simulink model "lqi16_discreto"  (R2025b)
settings: Solver=VariableStepAuto  StartTime=0.0  StopTime=10  RelTol=1e-3
values from neighbouring files (symbols this model uses):
  Cm = [1 0 0 0 0 0 0 0 0 0 1 0 ... (108 elements, 9x12)]    [parametros_LQI.mat]
  K = [8.61388977208e-09 -3.23938755891e-11 27.1624608635 1.22408347835e-11 5.15548702544e-09 -26.9052309444 4.91703547324e-11 2.27757364143e-13 56.1282376315 -9.6103215742e-14 8.73666069887e-14 -5.56559839576e-15 ... (64 elements, 4x16)]    [parametros_LQI.mat]
undefined symbols (not defined in the file or in its folder): C, L, sys
settings Model: Creator=rel  LastModifiedBy=rel

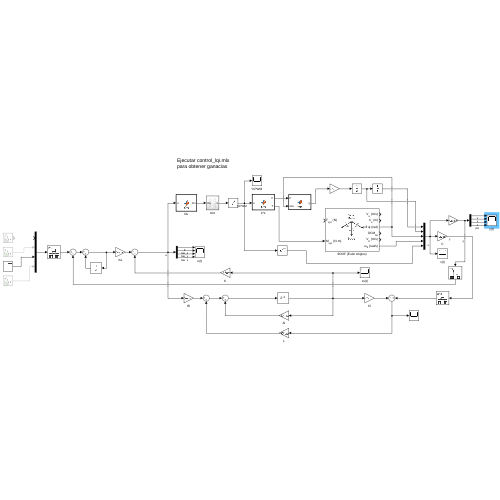
[thumbnail: Simulink's stored preview of the top-level diagram]
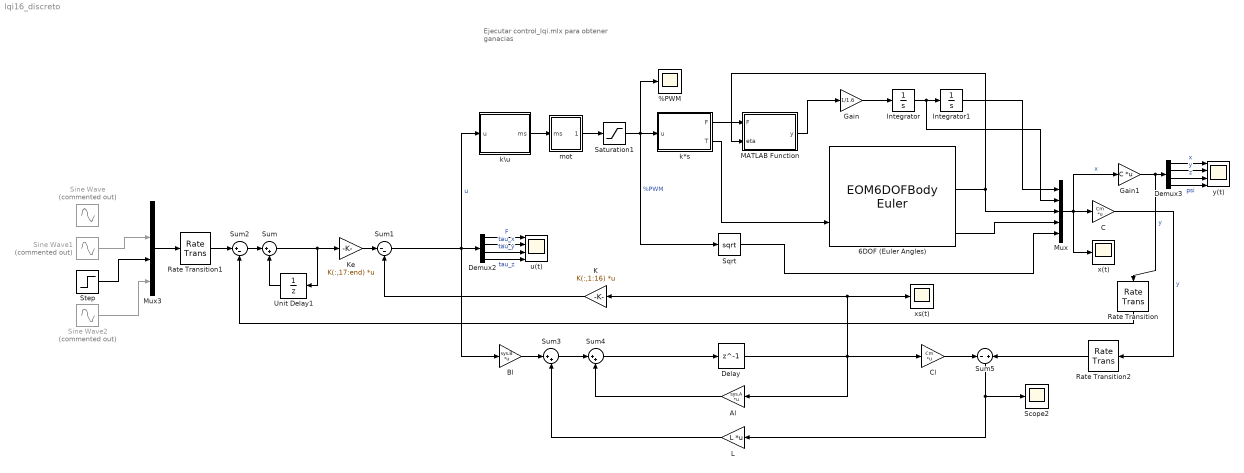
== system lqi16_discreto ==
  note: Ejecutar control_lqi.mlx
      | para obtener ganacias
  %PWM : Scope
      settings: ActiveDisplayYMinimum=-1  ActiveDisplayYMaximum=1  DataLoggingVariableName=ScopeData4
  6DOF (Euler Angles) : EOM6DOFBodyEuler  mass_0=1.6  inertia=diag([0.021915027 0.022124548 0.042349865])
  Al : Gain  Gain=sys.A  Multiplication=Matrix(K*u) (u vector)
  Bl : Gain  Gain=sys.B  Multiplication=Matrix(K*u) (u vector)
  C : Gain  Gain=Cm  Multiplication=Matrix(K*u) (u vector)
  Cl : Gain  Gain=Cm  Multiplication=Matrix(K*u)
  Delay : Delay  DelayLength=1
  Demux2 : Demux
  Demux3 : Demux
  Gain : Gain  Gain=1/1.6
  Gain1 : Gain  Gain=C  Multiplication=Matrix(K*u) (u vector)
  Integrator : Integrator
  Integrator1 : Integrator
  K : Gain  Gain=K(:,1:16)  Multiplication=Matrix(K*u) (u vector)
  Ke : Gain  Gain=K(:,17:end)  Multiplication=Matrix(K*u) (u vector)
  L : Gain  Gain=L  Multiplication=Matrix(K*u) (u vector)
  MATLAB Function : MATLAB Function  TreatAsAtomicUnit=on
  Mux : Mux  Inputs=5
  Mux3 : Mux
  Rate Transition : RateTransition  OutPortSampleTime=1/100
  Rate Transition1 : RateTransition  OutPortSampleTime=1/100
  Rate Transition2 : RateTransition  OutPortSampleTime=1/100
  Saturation1 : Saturate  UpperLimit=1  LowerLimit=0
  Scope2 : Scope
      settings: ActiveDisplayYMinimum=-1  ActiveDisplayYMaximum=1  DataLoggingVariableName=ScopeData6
  Sine Wave : Sin  Commented=on  Amplitude=0.5  Bias=1  Frequency=2  SampleTime=0
  Sine Wave1 : Sin  Commented=on  Amplitude=0.3  Frequency=3  SampleTime=0
  Sine Wave2 : Sin  Commented=on  SampleTime=0
  Sqrt : Sqrt
  Step : Step  SampleTime=0
  Sum : Sum  Inputs=|++
  Sum1 : Sum  Inputs=|--
  Sum2 : Sum  Inputs=|+-
  Sum3 : Sum  Inputs=|++
  Sum4 : Sum  Inputs=|++
  Sum5 : Sum  Inputs=-|+
  Unit Delay1 : UnitDelay  SampleTime=1/100  HasFrameUpgradeWarning=on
  k*s : MATLAB Function  TreatAsAtomicUnit=on
  k\u : MATLAB Function  TreatAsAtomicUnit=on
  mot : Subsystem
  u(t) : Scope  NumInputPorts=4
      settings: ActiveDisplayYMinimum=-47.245581502984457  ActiveDisplayYMaximum=52.593265856388996
  x(t) : Scope
      settings: ActiveDisplayYMinimum=-6.1052768376848006  ActiveDisplayYMaximum=6.0749182298943305  DataLoggingVariableName=ScopeData3
  xs(t) : Scope
      settings: ActiveDisplayYMinimum=-1  ActiveDisplayYMaximum=1  DataLoggingVariableName=ScopeData7
  y(t) : Scope  NumInputPorts=4
      settings: ActiveDisplayYMinimum=-326.12791447062108  ActiveDisplayYMaximum=63.895398333453315
  wires:
  Gain1/1 -> Rate Transition/1, Demux3/1  "y"
  K/1 -> Sum1/2
  Sum/1 -> Ke/1, Unit Delay1/1
  6DOF (Euler Angles)/3 -> MATLAB Function/2(eta), Mux/3
  mot/1(Out1) -> Saturation1/1
  k\u/1(ms) -> mot/1(ms)
  Saturation1/1 -> Sqrt/1, %PWM/1, k*s/1(u)  "%PWM"
  k*s/2(T) -> 6DOF (Euler Angles)/2
  k*s/1(F) -> MATLAB Function/1(F)
  Bl/1 -> Sum3/1
  Sum3/1 -> Sum4/1
  Cl/1 -> Sum5/1
  Al/1 -> Sum4/2
  L/1 -> Sum3/2
  Sum5/1 -> L/1, Scope2/1
  Integrator/1 -> Mux/2, Integrator1/1
  6DOF (Euler Angles)/6 -> Mux/4
  Mux/1 -> Gain1/1, x(t)/1, C/1  "x"
  Unit Delay1/1 -> Sum/2
  Sum2/1 -> Sum/1
  Ke/1 -> Sum1/1
  Mux3/1 -> Rate Transition1/1
  Sum1/1 -> Bl/1, Demux2/1, k\u/1(u)  "u"
  Sine Wave1/1 -> Mux3/2
  Sine Wave2/1 -> Mux3/4
  Demux2/1 -> u(t)/1  "F"
  Demux2/2 -> u(t)/2  "tau_x"
  Demux2/3 -> u(t)/3  "tau_y"
  Demux2/4 -> u(t)/4  "tau_z"
  Demux3/1 -> y(t)/1  "x"
  Demux3/2 -> y(t)/2  "y"
  Demux3/3 -> y(t)/3  "z"
  Demux3/4 -> y(t)/4  "psi"
  Sum4/1 -> Delay/1
  Gain/1 -> Integrator/1
  MATLAB Function/1(y) -> Gain/1
  Rate Transition/1 -> Sum2/2
  Rate Transition1/1 -> Sum2/1
  Integrator1/1 -> Mux/1
  Delay/1 -> xs(t)/1, K/1, Al/1, Cl/1
  Step/1 -> Mux3/3
  C/1 -> Rate Transition2/1  "y"
  Sqrt/1 -> Mux/5
  Rate Transition2/1 -> Sum5/2

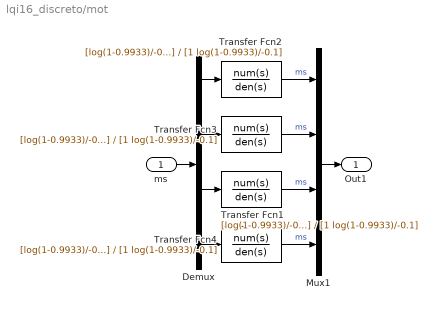
== system lqi16_discreto/mot ==
  ms : Inport
  Demux : Demux
  Mux1 : Mux
  Transfer Fcn{1..4} (4 alike) : TransferFcn  Numerator=[log(1-0.9933)/-0.1]  Denominator=[1 log(1-0.9933)/-0.1]
  Out1 : Outport
  wires:
  Transfer Fcn3/1 -> Mux1/2  "ms"
  Transfer Fcn1/1 -> Mux1/3  "ms"
  Demux/3 -> Transfer Fcn1/1
  Transfer Fcn4/1 -> Mux1/4  "ms"
  Demux/4 -> Transfer Fcn4/1
  Mux1/1 -> Out1/1
  Transfer Fcn2/1 -> Mux1/1  "ms"
  Demux/2 -> Transfer Fcn3/1
  Demux/1 -> Transfer Fcn2/1
  ms/1 -> Demux/1

== matlab function lqi16_discreto/k\u ==
  data: u input; ms output
function ms = fcn(u)
% L = 0.0080;
% kF = 0.1600*9.81;
% kM = 0.0086;
L = 0.268554;
kF = 7.965;
kM = 0.2;
A = [kF kF kF kF; -L*kF -L*kF L*kF L*kF; L*kF -L*kF -L*kF L*kF; -kM kM -kM kM];
ms = A\[u(1)+1.6*9.81; u(2:end)];

== matlab function lqi16_discreto/MATLAB Function ==
  data: F input; y output; eta input
function y = fcn(F, eta)
phi = eta(1);
theta = eta(2);
psi = eta(3);
y = [0;0;-1.6*9.81] + [sin(theta)*cos(psi) + sin(phi)*cos(theta)*sin(psi); ...
                    sin(theta)*sin(psi) - sin(phi)*cos(theta)*cos(psi); ...
                    cos(phi)*cos(theta)]*F;

== matlab function lqi16_discreto/k*s ==
  data: u input; F output; T output
function [F, T] = fcn(u)
% L = 0.0080;
% kF = 0.1600*9.81;
% kM = 0.0086;
L = 0.268554;
kF = 7.965;
kM = 0.2;
A = [kF kF kF kF; -L*kF -L*kF L*kF L*kF; L*kF -L*kF -L*kF L*kF; -kM kM -kM kM];
y = A*u;
F = y(1);
T = y(2:end);
